simulink model "diff_eq_filter"  (R2020b)
settings: Solver=VariableStepAuto  StartTime=0.0  StopTime=10.0  RelTol=1e-3
settings Model: Creator=shraddha  LastModifiedBy=shraddha

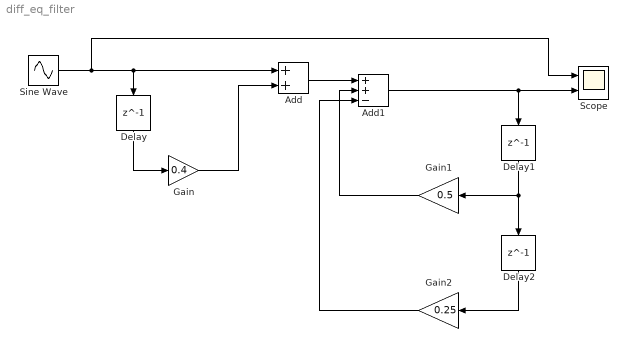
== system diff_eq_filter ==
  Add : Sum
  Add1 : Sum  Inputs=++-
  Delay : Delay  DelayLength=1
  Delay1 : Delay  DelayLength=1
  Delay2 : Delay  DelayLength=1
  Gain : Gain  Gain=0.4
  Gain1 : Gain  Gain=0.5
  Gain2 : Gain  Gain=0.25
  Scope : Scope  NumInputPorts=2
  Sine Wave : Sin  SampleTime=0
  wires:
  Sine Wave/1 -> Scope/1, Add/1, Delay/1
  Delay/1 -> Gain/1
  Gain/1 -> Add/2
  Delay2/1 -> Gain2/1
  Delay1/1 -> Delay2/1, Gain1/1
  Add/1 -> Add1/1
  Gain1/1 -> Add1/2
  Gain2/1 -> Add1/3
  Add1/1 -> Delay1/1, Scope/2
